simulink model "espaco_estados"  (Simulink 8.3)
settings: Solver=ode45  StartTime=0.0  StopTime=100.0  RelTol=1e-3
undefined symbols (not defined in the file): Rows
libraries: dspsigops x1, dspsrcs4 x1, simulink x1
settings Model: Creator=Jônatas  LastModifiedBy=Jônatas
settings DataIOCC: SignalLoggingSaveFormat=Dataset
settings DebuggingCC: UnderspecifiedInitializationDetection=Simplified  StateNameClashWarn=none
settings GRTTargetCC: CombineOutputUpdateFcns=on  GRTInterface=off

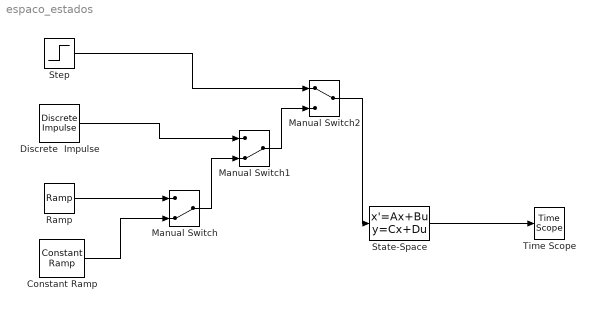
== system espaco_estados ==
  Constant Ramp : dspsigops/Constant Ramp  L=Rows  dim=1  Slope=1  dataType=Same as input  isSigned=on  wordLen=16  udDataType=sfix(16)  fracBitsMode=Best precision  numFracBits=15  Offset=0
  Discrete  Impulse : dspsrcs4/Discrete  Impulse  Delay=0  SampleTime=1  FrameSample=1  dataType=double  isSigned=on  wordLen=16  udDataType=sfix(16)  fracBitsMode=Best precision  numFracBits=15  OutDataTypeStr=double  LastOutDataTypeStr=double
  Manual Switch : ManualSwitch  CurrentSetting=0
  Manual Switch1 : ManualSwitch  CurrentSetting=0
  Manual Switch2 : ManualSwitch
  Ramp : simulink/Sources/Ramp  slope=1  start=0  X0=0
  State-Space : StateSpace  A=[0 0 0;1 0 -3;0 1 -3.5]  B=[0;0;1]  C=[75 90 15]  D=[0]  X0=0
  Step : Step  SampleTime=0
  Time Scope : TimeScope  DefaultConfigurationName=spbscopes.TimeScopeBlockCfg  ScopeSpecification=DataTag0
  wires:
  Ramp/1 -> Manual Switch/1
  Constant Ramp/1 -> Manual Switch/2
  Manual Switch/1 -> Manual Switch1/2
  Discrete  Impulse/1 -> Manual Switch1/1
  Step/1 -> Manual Switch2/1
  Manual Switch1/1 -> Manual Switch2/2
  Manual Switch2/1 -> State-Space/1
  State-Space/1 -> Time Scope/1
